simulink model "sampleModel1655_4_sub_sub"  (R2023a)
settings: Solver=VariableStepAuto  StartTime=0.0  StopTime=10.0  RelTol=1e-3
libraries: hdlsllib x2, simulink x1
settings Model: Creator=user1  LastModifiedBy=user1

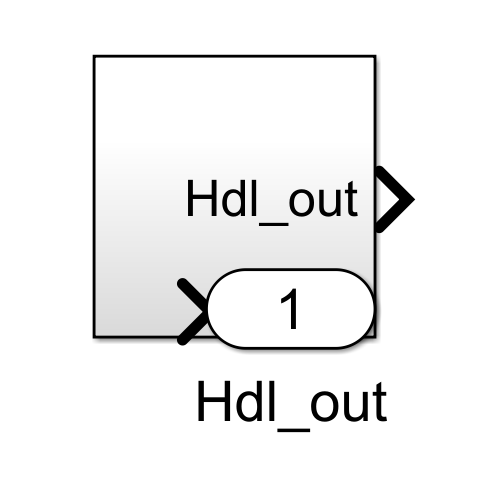
[thumbnail: Simulink's stored preview of the top-level diagram]
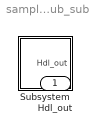
== system sampleModel1655_4_sub_sub ==
  Subsystem : Subsystem
  Hdl_out : Outport  OutDataTypeStr=uint8

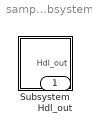
== system sampleModel1655_4_sub_sub/Subsystem ==
  Subsystem : Subsystem
  Hdl_out : Outport  OutDataTypeStr=uint8

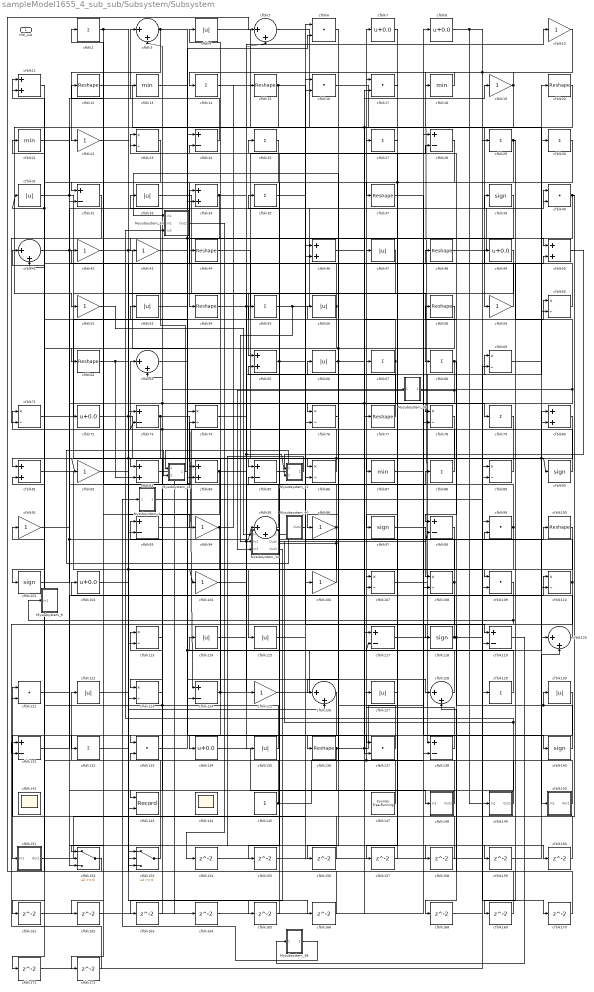
== system sampleModel1655_4_sub_sub/Subsystem/Subsystem ==
  Mysubsystem_14 : Subsystem  TreatAsAtomicUnit=on  RTWFcnName=Mysubsystem_14
      settings: RTWFcnNameOpts=User specified  RTWFileNameOpts=Use function name
  Mysubsystem_18 : Subsystem  TreatAsAtomicUnit=on  RTWFcnName=Mysubsystem_18
      settings: RTWFcnNameOpts=User specified  RTWFileNameOpts=Use function name
  Mysubsystem_26 : Subsystem  TreatAsAtomicUnit=on  RTWFcnName=Mysubsystem_26
      settings: RTWFcnNameOpts=User specified  RTWFileNameOpts=Use function name
  Mysubsystem_31 : Subsystem  TreatAsAtomicUnit=on  RTWFcnName=Mysubsystem_31
      settings: RTWFcnNameOpts=User specified  RTWFileNameOpts=Use function name
  Mysubsystem_33 : Subsystem  TreatAsAtomicUnit=on  RTWFcnName=Mysubsystem_33
      settings: RTWFcnNameOpts=User specified  RTWFileNameOpts=Use function name
  Mysubsystem_38 : Subsystem  TreatAsAtomicUnit=on  RTWFcnName=Mysubsystem_38
      settings: RTWFcnNameOpts=User specified  RTWFileNameOpts=Use function name
  Mysubsystem_4 : Subsystem  TreatAsAtomicUnit=on  RTWFcnName=Mysubsystem_4
      settings: RTWFcnNameOpts=User specified  RTWFileNameOpts=Use function name
  Mysubsystem_40 : Subsystem  TreatAsAtomicUnit=on  RTWFcnName=Mysubsystem_40
      settings: RTWFcnNameOpts=User specified  RTWFileNameOpts=Use function name
  Mysubsystem_9 : Subsystem  TreatAsAtomicUnit=on  RTWFcnName=Mysubsystem_9
      settings: RTWFcnNameOpts=User specified  RTWFileNameOpts=Use function name
  cfblk{10,19,22,42..43,52,59,82,91,94,96,104,106,125} (14 alike) : Gain  OutDataTypeStr=uint8
  cfblk{12,15,20,37,44,48,54,58,62,77,100,136} (12 alike) : Reshape
  cfblk{39,90,97,101,118,140} (6 alike) : Signum
  cfblk{7..8,49,72,102,134} (6 alike) : Bias  Bias=0.0  SaturateOnIntegerOverflow=off
  cfblk{23,60,69,71,74,76,78,86,89,107..108,110,113,123} (14 alike) : Product  Inputs=*/  OutDataTypeStr=uint8  RndMeth=Zero  SaturateOnIntegerOverflow=on
  cfblk{6,16..17,40,99,109,121,133,137} (9 alike) : DotProduct  OutDataTypeStr=uint8
  cfblk{11,34,46,50,65,80..81,83..84} (9 alike) : Sum  OutDataTypeStr=uint8
  cfblk{4,31,33,47,53,56,66,114..115,122,127,130,135} (13 alike) : Abs  OutDataTypeStr=uint8  SaturateOnIntegerOverflow=off
  cfblk{24,28,32,73,85,93,98,117,119,124,131,138} (12 alike) : Sum  Inputs=+-  OutDataTypeStr=uint8
  cfblk{3,5,41,63,95,120,126,128} (8 alike) : Sum  Inputs=|++  OutDataTypeStr=uint8
  cfblk{2,14,25,27,29..30,35,55,67..68,79,88,129,132} (14 alike) : Sum  Inputs=+  OutDataTypeStr=uint8
  cfblk{13,18,21,87} (4 alike) : MinMax  OutDataTypeStr=uint8
  cfblk141 : Scope
      settings: Floating=on
  cfblk143 : Record  FileSettingsInternal="{\"entries\":[{\"content\":{\"excelSettings\":{\"content\":{},\"type\":\"Streamout.ExcelSettings\"}},\"type\":\"Streamout.FileSettingStorage\",\"uuid\":\"\"}],\"packageUris\":[\"http:\\/\\/schema.mathworks.com\\/mf0\\/streamout_blocks\\/R2020a\"],\"version\":\"1.0\"}"  Layout=[1 1]  SignalsInternal="{\"entries\":[{\"content\":{\"signals\":[{\"content\":{\"blockPath\":[],\"dimensions\":[1],\"domain\":\"\",\"lineColor\":\"#a2142f\",\"plots\":[1],\"port\":1,\"signalID\":31664,\"signalName\":\"cfblk126\"},\"type\":\"RecordBlkView.Signal\",\"uuid\":\"\"},{\"content\":{\"blockPath\":[],\"dimensions\":[1],\"domain\":\"\",\"lineColor\":\"#139fff\",\"plots\":[1],\"port\":2,\"signalID\":31667,\"signalName\":\"cfblk49\"},\"type\":\"RecordBlkView.Signal\",\"uuid\":\"\"}]},\"type\":\"RecordBlkView.InputSignals\",\"uuid\":\"\"}],\"packageUris\":[\"http:\\/\\/schema.mathworks.com\\/mf0\\/streamout_blocks\\/R2020a\"],\"version\":\"1.0\"}"  VisualizationBindings="{\"xyplotplugin\":{\"info\":[{\"series\":[{\"bindingParametersList\":[{\"parameter\":\"X-Axis\",\"signalID\":31664,\"signalName\":\"cfblk126\"},{\"parameter\":\"Y-Axis\",\"signalID\":31667,\"signalName\":\"cfblk49\"}],\"seriesID\":51804}],\"subplotID\":1}]}}"  CompatibilityTag=XY  st=-1
  cfblk144 : Scope
      settings: Floating=on
  cfblk145 : Constant  OutDataTypeStr=uint8  SampleTime=-1
  cfblk147 : hdlsllib/Sources/Counter Free-Running  NumBits=16  tsamp=-1
  cfblk148 : Subsystem
      settings: LibrarySourceBlock=|
      | hdlsllib/Ports &
      | Subsystems/Subsystem
  cfblk149 : Subsystem
      settings: LibrarySourceBlock=|
      | hdlsllib/Ports &
      | Subsystems/Subsystem
  cfblk150 : Subsystem
      settings: LibrarySourceBlock=|
      | hdlsllib/Ports &
      | Subsystems/Subsystem
  cfblk151 : Subsystem
      settings: LibrarySourceBlock=|
      | hdlsllib/Ports &
      | Subsystems/Subsystem
  cfblk152 : Switch  OutDataTypeStr=uint8  SaturateOnIntegerOverflow=off  InputSameDT=off
  cfblk153 : Switch  OutDataTypeStr=uint8  SaturateOnIntegerOverflow=off  InputSameDT=off
  cfblk{154..166,168..172} (18 alike) : Delay  SampleTime=1
  Hdl_out : Outport  OutDataTypeStr=uint8
  wires:
  Mysubsystem_40/1(Out1) -> cfblk106/1
  Mysubsystem_38/1(Out1) -> Mysubsystem_4/1(In1)
  cfblk119/1 -> Mysubsystem_38/1(In1)
  Mysubsystem_33/1(Out1) -> cfblk154/1
  Mysubsystem_18/1(Out1) -> Mysubsystem_33/2(In2)
  Mysubsystem_31/1(Out1) -> cfblk158/1
  cfblk50/1 -> Mysubsystem_31/1(In1)
  Mysubsystem_26/1(Out1) -> cfblk49/1, Mysubsystem_26/1(In1), cfblk152/2
  Mysubsystem_14/1(Out1) -> Mysubsystem_18/2(In2)
  cfblk85/1 -> Mysubsystem_18/1(In1)
  Mysubsystem_14/3(Out3) -> cfblk163/1
  cfblk52/1 -> Mysubsystem_14/1(In1)
  Mysubsystem_14/2(Out2) -> Mysubsystem_33/3(In3), cfblk162/1
  Mysubsystem_4/1(Out1) -> cfblk89/2
  cfblk172/1 -> cfblk131/1
  cfblk171/1 -> cfblk69/2
  cfblk170/1 -> cfblk128/2
  cfblk169/1 -> cfblk11/2
  cfblk100/1 -> cfblk169/1
  cfblk168/1 -> cfblk99/1
  cfblk166/1 -> cfblk73/1
  cfblk165/1 -> cfblk65/2
  cfblk102/1 -> cfblk165/1
  cfblk164/1 -> cfblk138/2
  cfblk163/1 -> cfblk133/2
  cfblk162/1 -> cfblk108/2
  cfblk161/1 -> cfblk17/2
  cfblk32/1 -> cfblk161/1
  cfblk160/1 -> cfblk28/1
  cfblk159/1 -> cfblk120/2
  cfblk121/1 -> cfblk159/1
  cfblk158/1 -> cfblk117/1
  cfblk157/1 -> cfblk107/2
  cfblk27/1 -> cfblk157/1
  cfblk156/1 -> cfblk81/2
  cfblk6/1 -> cfblk156/1
  cfblk155/1 -> cfblk16/2
  cfblk154/1 -> cfblk89/1
  cfblk74/1 -> cfblk86/2
  cfblk77/1 -> cfblk55/1
  cfblk91/1 -> cfblk40/2
  cfblk49/1 -> cfblk143/2
  cfblk17/1 -> cfblk97/1
  cfblk80/1 -> cfblk153/2, cfblk110/2
  cfblk14/1 -> cfblk80/2
  cfblk135/1 -> cfblk21/1, cfblk53/1
  cfblk99/1 -> cfblk3/2, cfblk73/2, cfblk126/1
  cfblk96/1 -> cfblk44/1, cfblk153/3
  cfblk153/1 -> cfblk91/1
  cfblk145/1 -> cfblk8/1, cfblk63/2
  cfblk127/1 -> cfblk47/1
  cfblk131/1 -> cfblk107/1
  cfblk122/1 -> cfblk48/1
  cfblk28/1 -> cfblk41/2
  cfblk151/1(Out1) -> cfblk46/2
  cfblk84/1 -> cfblk135/1, cfblk152/1
  cfblk23/1 -> cfblk62/1
  cfblk67/1 -> cfblk41/1, cfblk96/1
  cfblk66/1 -> Mysubsystem_33/1(In1), cfblk19/1
  cfblk11/1 -> cfblk101/1
  cfblk152/1 -> cfblk5/1
  cfblk101/1 -> cfblk84/1, cfblk95/1
  cfblk125/1 -> cfblk80/1
  cfblk53/1 -> cfblk39/1
  cfblk86/1 -> cfblk82/1, cfblk2/1
  cfblk89/1 -> cfblk81/1
  cfblk87/1 -> cfblk109/2
  cfblk136/1 -> cfblk110/1, cfblk60/1, cfblk152/3
  cfblk93/1 -> cfblk6/1
  cfblk12/1 -> cfblk46/1
  cfblk124/1 -> cfblk88/1, cfblk4/1
  cfblk41/1 -> cfblk125/1, cfblk50/2
  cfblk63/1 -> cfblk128/1
  cfblk132/1 -> cfblk153/1
  cfblk30/1 -> cfblk87/1, cfblk155/1
  cfblk82/1 -> cfblk113/2
  cfblk113/1 -> cfblk23/2
  cfblk24/1 -> cfblk3/1
  cfblk13/1 -> cfblk78/1
  cfblk34/1 -> cfblk10/1, cfblk43/1
  cfblk37/1 -> cfblk140/1
  cfblk134/1 -> cfblk148/1(In1)
  cfblk39/1 -> cfblk124/2, cfblk71/2
  cfblk97/1 -> cfblk108/1
  cfblk81/1 -> cfblk129/1
  cfblk133/1 -> cfblk117/2, cfblk6/2
  cfblk55/1 -> Mysubsystem_14/2(In2), cfblk20/1
  cfblk18/1 -> cfblk14/1
  cfblk22/1 -> cfblk93/2, cfblk90/1
  cfblk21/1 -> cfblk72/1
  cfblk126/1 -> cfblk143/1
  cfblk118/1 -> cfblk58/1, cfblk170/1, cfblk66/1
  cfblk4/1 -> cfblk150/1(In1)
  cfblk120/1 -> cfblk35/1
  cfblk71/1 -> cfblk34/2
  cfblk8/1 -> cfblk29/1, cfblk149/1(In1)
  cfblk65/1 -> cfblk25/1, cfblk118/1
  cfblk76/1 -> cfblk136/1
  cfblk78/1 -> cfblk134/1
  cfblk117/1 -> cfblk30/1
  cfblk33/1 -> cfblk68/1
  cfblk140/1 -> cfblk24/2, cfblk130/1
  cfblk35/1 -> cfblk16/1
  cfblk7/1 -> cfblk37/1
  cfblk115/1 -> cfblk100/1
  cfblk147/1 -> cfblk113/1
  cfblk95/1 -> cfblk74/2, cfblk12/1
  cfblk42/1 -> cfblk74/1, cfblk166/1
  cfblk83/1 -> cfblk137/1, cfblk164/1
  cfblk123/1 -> cfblk33/1
  cfblk20/1 -> cfblk32/2
  cfblk150/1(Out1) -> cfblk93/1
  cfblk2/1 -> cfblk32/1, cfblk126/2
  cfblk114/1 -> cfblk69/1, cfblk98/2
  cfblk94/1 -> cfblk133/1, cfblk15/1
  cfblk109/1 -> Mysubsystem_9/1(In1), cfblk131/2
  cfblk108/1 -> cfblk121/2, cfblk42/1
  cfblk19/1 -> cfblk123/2, cfblk137/2, cfblk18/1
  cfblk46/1 -> cfblk127/1, cfblk78/2
  cfblk137/1 -> cfblk102/1
  cfblk59/1 -> cfblk11/1, cfblk31/1
  cfblk79/1 -> cfblk123/1
  cfblk47/1 -> cfblk65/1
  cfblk54/1 -> cfblk28/2, cfblk79/1
  cfblk106/1 -> cfblk85/2, cfblk95/2
  cfblk88/1 -> cfblk63/1
  cfblk5/1 -> cfblk77/1
  cfblk3/1 -> cfblk22/1, cfblk50/1
  cfblk43/1 -> cfblk24/1
  cfblk15/1 -> cfblk52/1, cfblk119/1
  cfblk129/1 -> cfblk114/1
  cfblk29/1 -> cfblk109/1, cfblk84/2
  cfblk60/1 -> cfblk34/1
  cfblk58/1 -> cfblk132/1, cfblk76/1
  cfblk62/1 -> cfblk104/1, cfblk160/1, cfblk83/2
  cfblk130/1 -> cfblk151/1(In1)
  cfblk69/1 -> cfblk120/1
  cfblk10/1 -> cfblk138/1, cfblk119/2
  cfblk16/1 -> cfblk59/1
  cfblk72/1 -> cfblk85/1, cfblk94/1
  cfblk40/1 -> cfblk121/1, cfblk60/2
  cfblk25/1 -> cfblk54/1
  cfblk68/1 -> Mysubsystem_14/3(In3), cfblk76/2, cfblk98/1
  cfblk98/1 -> cfblk115/1
  cfblk104/1 -> Mysubsystem_31/2(In2), cfblk5/2
  cfblk90/1 -> cfblk27/1
  cfblk48/1 -> cfblk40/1
  cfblk73/1 -> cfblk124/1, cfblk172/1
  cfblk148/1(Out1) -> cfblk67/1, cfblk56/1
  cfblk56/1 -> cfblk23/1, cfblk171/1
  cfblk31/1 -> cfblk83/1, cfblk13/1
  cfblk138/1 -> cfblk17/1
  cfblk107/1 -> cfblk99/2
  cfblk149/1(Out1) -> cfblk122/1
  cfblk44/1 -> cfblk86/1
  cfblk110/1 -> cfblk71/1, cfblk168/1
  cfblk128/1 -> cfblk7/1

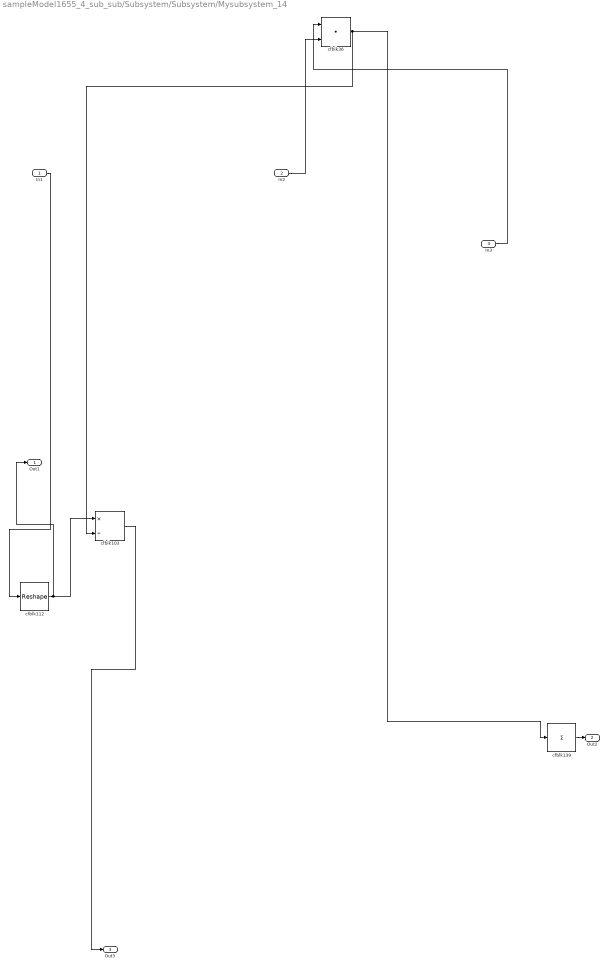
== system sampleModel1655_4_sub_sub/Subsystem/Subsystem/Mysubsystem_14 ==
  In1 : Inport
  In2 : Inport  Port=2
  In3 : Inport  Port=3
  cfblk103 : Product  Inputs=*/  RndMeth=Zero  SaturateOnIntegerOverflow=on
  cfblk112 : Reshape
  cfblk139 : Sum  Inputs=+
  cfblk36 : DotProduct  OutDataTypeStr=Inherit: Inherit via internal rule
  Out1 : Outport
  Out2 : Outport  Port=2
  Out3 : Outport  Port=3
  wires:
  cfblk139/1 -> Out2/1
  cfblk112/1 -> Out1/1, cfblk103/1
  In1/1 -> cfblk112/1
  cfblk36/1 -> cfblk139/1, cfblk103/2
  cfblk103/1 -> Out3/1
  In2/1 -> cfblk36/2
  In3/1 -> cfblk36/1

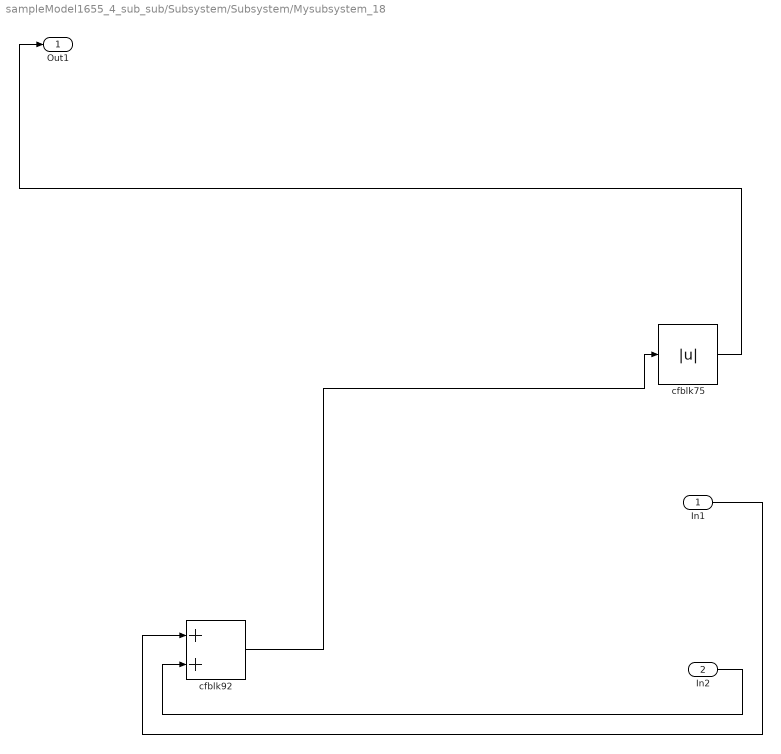
== system sampleModel1655_4_sub_sub/Subsystem/Subsystem/Mysubsystem_18 ==
  In1 : Inport
  In2 : Inport  Port=2
  cfblk75 : Abs  SaturateOnIntegerOverflow=off
  cfblk92 : Sum
  Out1 : Outport
  wires:
  cfblk92/1 -> cfblk75/1
  cfblk75/1 -> Out1/1
  In2/1 -> cfblk92/2
  In1/1 -> cfblk92/1

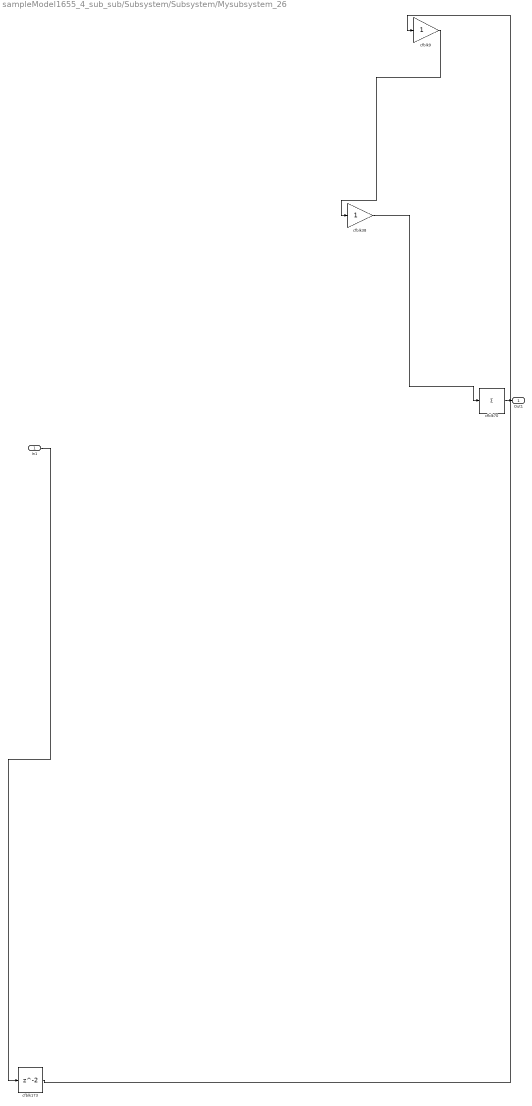
== system sampleModel1655_4_sub_sub/Subsystem/Subsystem/Mysubsystem_26 ==
  In1 : Inport
  cfblk173 : Delay  SampleTime=1
  cfblk38 : Gain
  cfblk70 : Sum  Inputs=+
  cfblk9 : Gain
  Out1 : Outport
  wires:
  cfblk38/1 -> cfblk70/1
  cfblk9/1 -> cfblk38/1
  cfblk173/1 -> cfblk9/1
  cfblk70/1 -> Out1/1
  In1/1 -> cfblk173/1

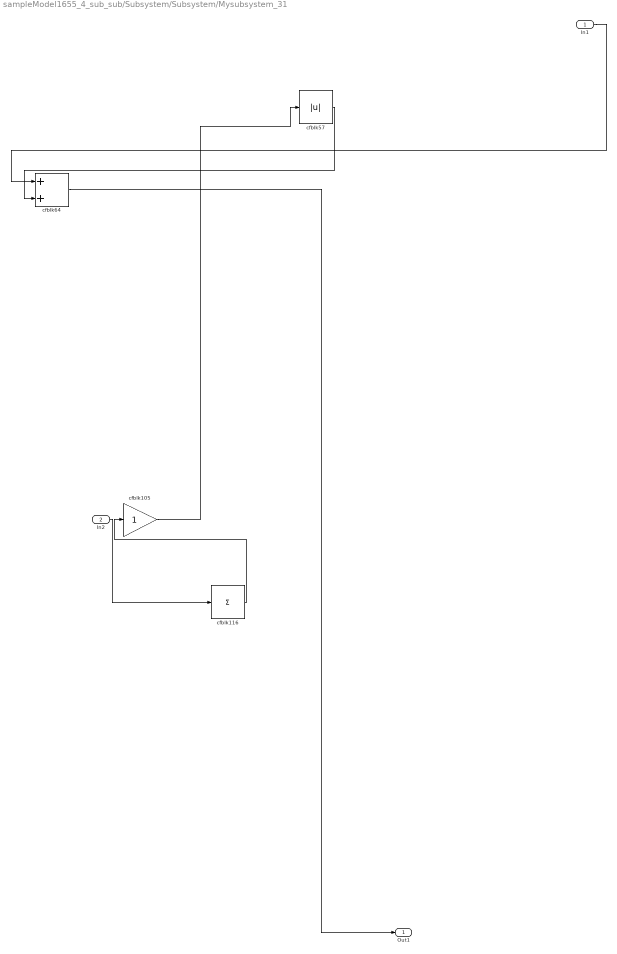
== system sampleModel1655_4_sub_sub/Subsystem/Subsystem/Mysubsystem_31 ==
  In1 : Inport
  In2 : Inport  Port=2
  cfblk105 : Gain
  cfblk116 : Sum  Inputs=+
  cfblk57 : Abs  SaturateOnIntegerOverflow=off
  cfblk64 : Sum
  Out1 : Outport
  wires:
  cfblk105/1 -> cfblk57/1
  cfblk116/1 -> cfblk105/1
  cfblk64/1 -> Out1/1
  cfblk57/1 -> cfblk64/2
  In1/1 -> cfblk64/1
  In2/1 -> cfblk116/1

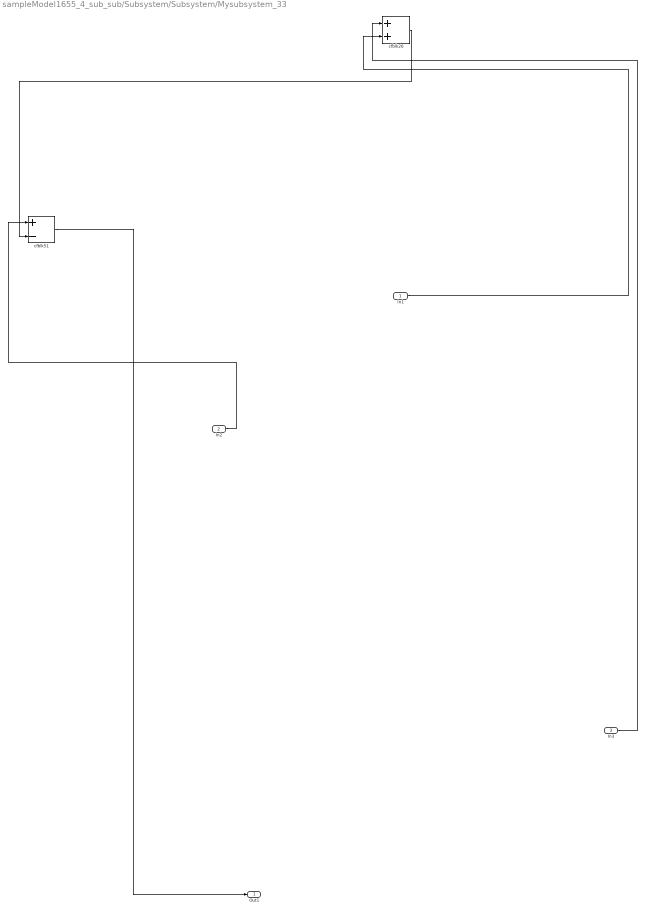
== system sampleModel1655_4_sub_sub/Subsystem/Subsystem/Mysubsystem_33 ==
  In1 : Inport
  In2 : Inport  Port=2
  In3 : Inport  Port=3
  cfblk26 : Sum
  cfblk51 : Sum  Inputs=+-
  Out1 : Outport
  wires:
  In3/1 -> cfblk26/1
  cfblk26/1 -> cfblk51/2
  In1/1 -> cfblk26/2
  In2/1 -> cfblk51/1
  cfblk51/1 -> Out1/1

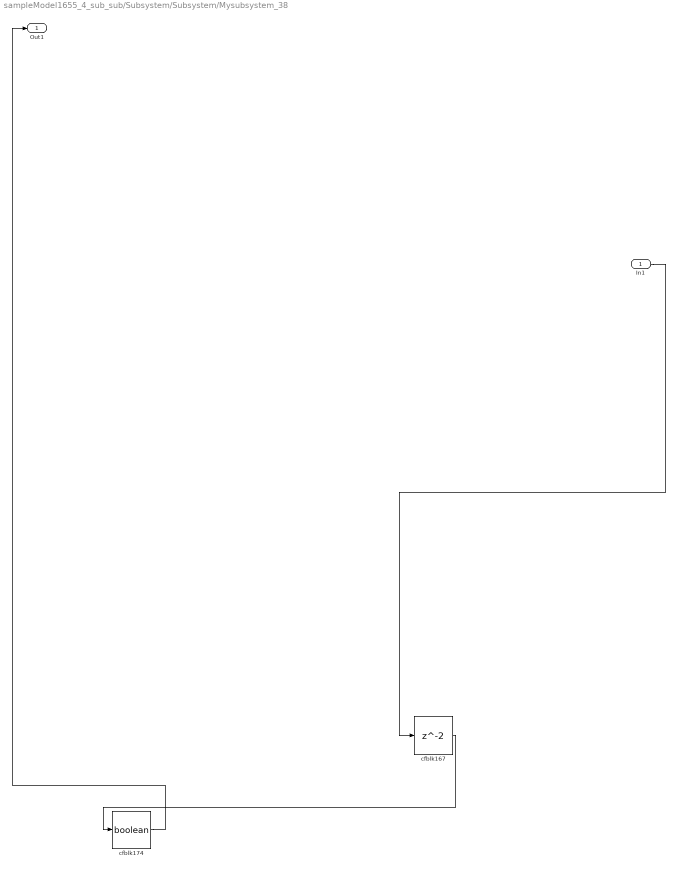
== system sampleModel1655_4_sub_sub/Subsystem/Subsystem/Mysubsystem_38 ==
  In1 : Inport
  cfblk167 : Delay  SampleTime=1
  cfblk174 : DataTypeConversion  OutDataTypeStr=boolean  SaturateOnIntegerOverflow=off  RndMeth=Floor
  Out1 : Outport
  wires:
  cfblk174/1 -> Out1/1
  cfblk167/1 -> cfblk174/1
  In1/1 -> cfblk167/1

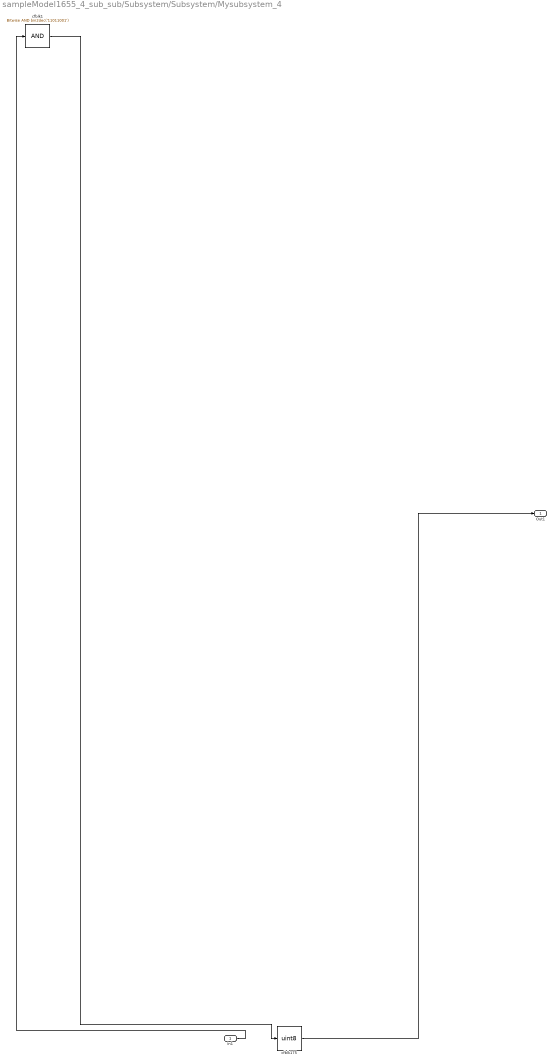
== system sampleModel1655_4_sub_sub/Subsystem/Subsystem/Mysubsystem_4 ==
  In1 : Inport
  cfblk1 : simulink/Logic and Bit Operations/Bitwise Operator  logicop=AND  UseBitMask=on  BitMask=bin2dec('11011001')  BitMaskRealWorld=Stored Integer
      settings: LibrarySourceBlock=|
      | hdlsllib/Logic and Bit
      | Operations/Bitwise
      | Operator
  cfblk175 : DataTypeConversion  OutDataTypeStr=uint8  SaturateOnIntegerOverflow=off  RndMeth=Floor
  Out1 : Outport
  wires:
  cfblk1/1 -> cfblk175/1
  cfblk175/1 -> Out1/1
  In1/1 -> cfblk1/1

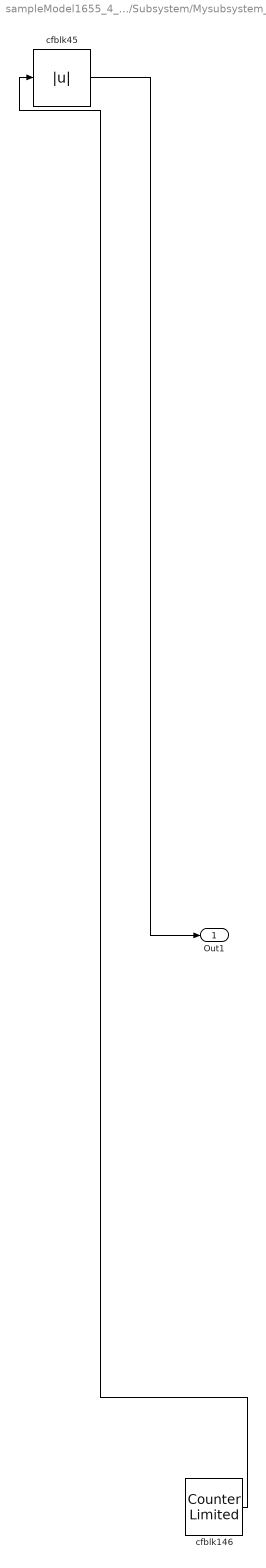
== system sampleModel1655_4_sub_sub/Subsystem/Subsystem/Mysubsystem_40 ==
  cfblk146 : hdlsllib/Sources/Counter Limited  uplimit=7  tsamp=-1
  cfblk45 : Abs  SaturateOnIntegerOverflow=off
  Out1 : Outport
  wires:
  cfblk146/1 -> cfblk45/1
  cfblk45/1 -> Out1/1

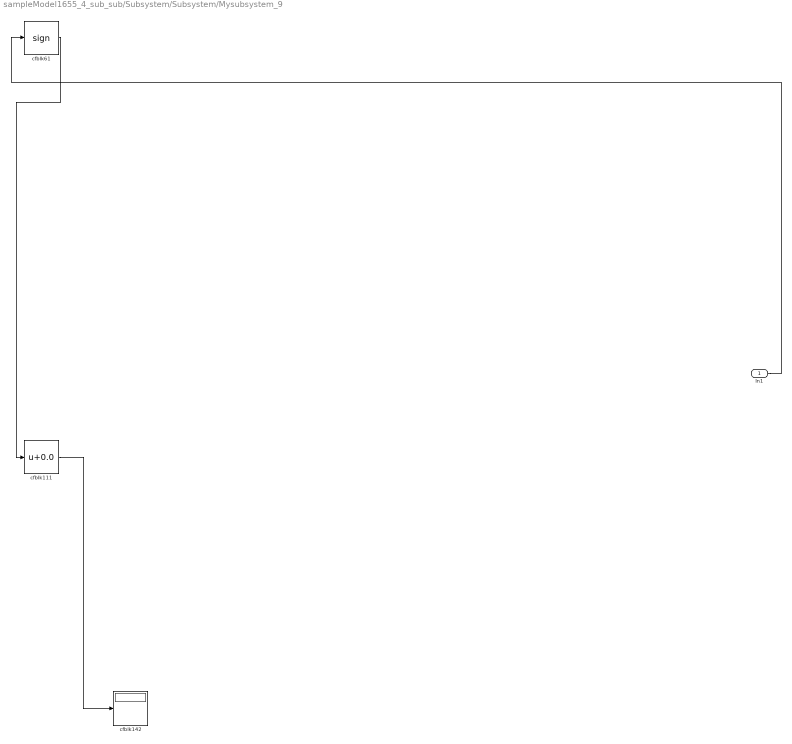
== system sampleModel1655_4_sub_sub/Subsystem/Subsystem/Mysubsystem_9 ==
  In1 : Inport
  cfblk111 : Bias  Bias=0.0  SaturateOnIntegerOverflow=off
  cfblk142 : Display
  cfblk61 : Signum
  wires:
  cfblk61/1 -> cfblk111/1
  cfblk111/1 -> cfblk142/1
  In1/1 -> cfblk61/1

== system sampleModel1655_4_sub_sub/Subsystem/Subsystem/cfblk148 ==
  In1 : Inport
  Out1 : Outport
  wires:
  In1/1 -> Out1/1

== system sampleModel1655_4_sub_sub/Subsystem/Subsystem/cfblk149 ==
  In1 : Inport
  Out1 : Outport
  wires:
  In1/1 -> Out1/1

== system sampleModel1655_4_sub_sub/Subsystem/Subsystem/cfblk150 ==
  In1 : Inport
  Out1 : Outport
  wires:
  In1/1 -> Out1/1

== system sampleModel1655_4_sub_sub/Subsystem/Subsystem/cfblk151 ==
  In1 : Inport
  Out1 : Outport
  wires:
  In1/1 -> Out1/1
